simulink model "rx_channelizer_PL"  (R2024a)
settings: Solver=VariableStepAuto  StartTime=0.0  StopTime=num_ch*150/fs  RelTol=1e-3
PreLoadFcn:
  | ch_rate = 41e6; % per channel sample rate
  | num_ch = 32;
  | flip_cnt = num_ch/2 - 1; % flip data count size
  | % 6 coeffs/ch;
  | PLclk=ch_rate*16; % PL clock frequency
  | fs = ch_rate*num_ch;
  | sample_rate = 1/fs;
  | base_freq=1e6; % what base channel frequency to modulate?
  | 
  | generate_prototype_FIR; % create FIR coeffs
undefined symbols (not defined in the file): ch0, ch1, ch10, ch11, ch12, ch13, ch14, ch15, ch16, ch17, ch18, ch19, ch2, ch20, ch21, ch22, ch23, ch24, ch25, ch26, ch27, ch28, ch29, ch3, ch30, ch31, ch4, ch5, ch6, ch7, ch8, ch9, S, vsva2197, xcvc1902
libraries: hdlBasic x69, dspsrcs4 x4, hdlSSR x3, hdlDSPIP x2, dspmlti4 x1, dspxfrm3 x1, vmcUtilities x1
(part 1 of 2)
settings Model: Creator=mmi  LastModifiedBy=robg
settings SolverCC: AlgebraicLoopSolver=TrustRegion
settings DebuggingCC: UnconnectedInputMsg=warning  UnconnectedOutputMsg=warning  UnconnectedLineMsg=warning
settings HardwareCC: ProdBitPerPointer=32  ProdBitPerSizeT=32  ProdBitPerPtrDiffT=32  ProdLargestAtomicFloat=None  ProdIntDivRoundTo=Undefined  ProdEndianess=Unspecified  ProdWordSize=32  ProdHWDeviceType=ASIC/FPGA->ASIC/FPGA  TargetBitPerLong=64  TargetBitPerPointer=64  TargetBitPerSizeT=64  TargetBitPerPtrDiffT=64  TargetLongLongMode=on  TargetIntDivRoundTo=Zero  TargetEndianess=LittleEndian  TargetWordSize=64  TargetHWDeviceType=Custom Processor->MATLAB Host Computer  ProdEqTarget=off
settings ModelReferenceCC: EnableRefExpFcnMdlSchedulingChecks=on
settings RTWCC: GPUComputeCapability=3.5  DLArmComputeVersion=19.05
settings ConfigComp: CovBoundaryAbsTol=1.0e-5

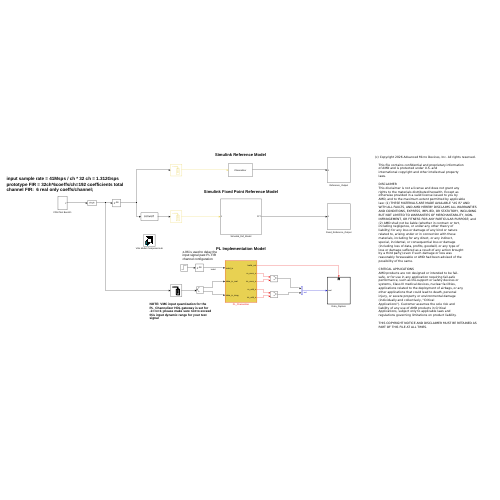
[thumbnail: Simulink's stored preview of the top-level diagram]
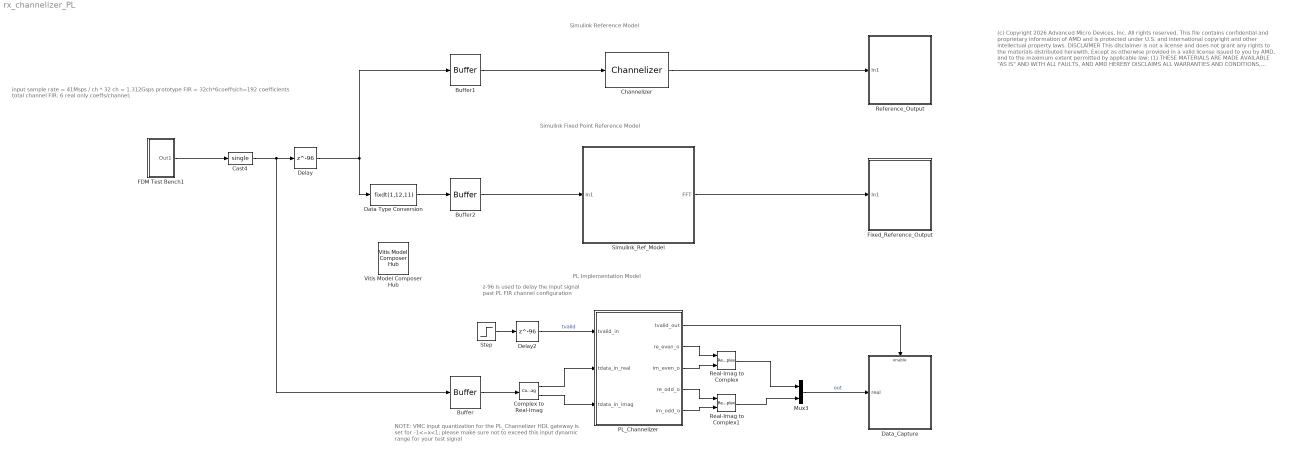
== system rx_channelizer_PL ==
  note: PL Implementation Model
  note: Simulink Fixed Point Reference Model
  note: Simulink Reference Model
  note: z-96 is used to delay the input signal past PL FIR channel configuration
  note: input sample rate = 41Msps / ch * 32 ch = 1.312Gsps
      | prototype FIR = 32ch*6coeffs/ch=192 coefficients total
      | channel FIR: 6 real only coeffs/channel;
  note: NOTE: VMC input quantization for the PL_Channelizer HDL gateway is set for -1<=x<1; please make sure not to exceed this input dynamic range for your test signal
  note: (c) Copyright 2026 Advanced Micro Devices, Inc. All rights reserved.
      |
      | This file contains confidential and proprietary information
      | of AMD and is protected under U.S. and
      | international copyright and other intellectual property
      | laws.
      |
      | DISCLAIMER
      | This disclaimer is not a license and does not grant any
      | rights to the materials distributed herewith. Except as
      | otherwise provided in a valid license issued to you by
      | AMD, and to the maximum extent permitted by applicable
      | law: (1) THESE MATERIALS ARE MADE AVAILABLE "AS IS" AND
      | WITH ALL FAULTS, AND AMD HEREBY DISCLAIMS ALL WARRANTIES
      | AND CONDITIONS, EXPRESS, IMPLIED, OR STATUTORY, INCLUDING
      | BUT NOT LIMITED TO WARRANTIES OF MERCHANTABILITY, NON-
      | INFRINGEMENT, OR FITNESS FOR ANY PARTICULAR PURPOSE; and
      | (2) AMD shall not be liable (whether in contract or tort,
      | including negligence, or under any other theory of
      | liability) for any loss or damage of any kind or nature
      | related to, arising under or in connection with these
      | materials, including for any direct, or any indirect,
      | special, incidental, or consequential loss or damage
      | (including loss of data, profits, goodwill, or any type of
      | loss or damage suffered as a result of any action brought
      | by a third party) even if such damage or loss was
      | reasonably foreseeable or AMD had been advised of the
      | possibility of the same.
      |
      | CRITICAL APPLICATIONS
      | AMD products are not designed or intended to be fail-
      | safe, or for use in any application requiring fail-safe
      | performance, such as life-support or safety devices or
      | systems, Class III medical devices, nuclear facilities,
      | applications related to the deployment of airbags, or any
      | other applications that could lead to death, personal
      | injury, or severe property or environmental damage
      | (individually and collectively, "Critical
      | Applications"). Customer assumes the sole risk and
      | liability of any use of AMD products in Critical
      | Applications, subject only to applicable laws and
      | regulations governing limitations on product liability.
      |
      | THIS COPYRIGHT NOTICE AND DISCLAIMER MUST BE RETAINED AS
      | PART OF THIS FILE AT ALL TIMES.
  Buffer : Buffer  N=2  OutputFrames=off
  Buffer1 : Buffer  N=num_ch*1  OutputFrames=off
  Buffer2 : Buffer  N=num_ch  OutputFrames=off
  Cast4 : DataTypeConversion  OutDataTypeStr=single  SaturateOnIntegerOverflow=off  RndMeth=Floor
  Channelizer : dspmlti4/Channelizer  NumFrequencyBands=32  DecimationFactor=Number of frequency bands  Specification=Coefficients  CoefficientsPort=off  NumTapsPerBand=6  StopbandAttenuation=80  LowpassCoefficients=pf  AllowArbitraryInputLength=off  BandsAsSeparateOutputPorts=off  SimulateUsing=Interpreted execution
  Complex to Real-Imag : ComplexToRealImag
  Data Type Conversion : DataTypeConversion  OutDataTypeStr=fixdt(1,12,11)  SaturateOnIntegerOverflow=off  RndMeth=Floor
  Data_Capture : Subsystem  TreatAsAtomicUnit=on
  Delay : Delay  DelayLength=96
  Delay2 : Delay  DelayLength=96
  FDM Test Bench1 : Subsystem
  Fixed_Reference_Output : Subsystem
  Mux3 : Mux  Inputs=2
  PL_Channelizer : Subsystem
  Real-Imag to Complex : RealImagToComplex
  Real-Imag to Complex1 : RealImagToComplex
  Reference_Output : Subsystem
  Simulink_Ref_Model : Subsystem
  Step : Step  Time=65/(ch_rate*16)  SampleTime=1/(ch_rate*16)
  Vitis Model Composer Hub : vmcUtilities/Vitis Model Composer Hub  Tag=genX  CodeGeneration=off  SubsystemName=PL_Channelizer  BlockHierPath=rx_channelizer_PL/PL_Channelizer  CompilationType=HDLCompilation  SubsystemType=HDLNode  ExportTypeV2=IP Catalog  StartColumn=1  NumberOfColumns=1  TargetDirectory=./netlist_PL  exportDesign=off  analyzeDesign=on  validateDesignOnHw=off  ExportType=AI Engines  IpVendor=xilinx.com  IpLibrary=hls  IpVersion=1.0  IpHWLanguage=Verilog  AieCompilerOptions={}  AieSimulatorOptions={}  CreateTestbench=on  TestbenchStackSize=10  RunRtlSim=off  RunCSim=off  RunAieSim=off  AieSimTimeout=50000  RunAieSimProfiling=off  LaunchVitisAnalyzer=off  PlotOutput=off  RunX86Sim=off  X86SimTimeout=10  GenHwImage=off  GenLibadfXo=on  GenHwValidationCode=off  PlatformType=Not Specified  HwSystemType=Baremetal  HwValidationTarget=hw  ProjDevice=Versal VCK190 Evaluation Platform with New SD Level Shifter (xcvc1902-vsva2197-2MP-e-S)  ProjDevicePart=xcvc1902-vsva2197-2MP-e-S  AIEType=AIE  SamplePeriod=-1  ClockFrequency=200  DataPathParallelism=1  xilinxfamily=versalaicore  part=xcvc1902  speed=-2MP-e-S  package=vsva2197  directory=./netlist_PL/ip/PL_Channelizer/src  testbench=off  incr_netlist=off  synthesis_tool=Vivado  clock_wrapper=Clock Enables  dbl_ovrd=According to Block Masks  dcm_input_clock_period=10  sysclk_period=1e9/PLclk  simulink_period=1/(ch_rate*16)  eval_field=0  IPInfoJsonString="{\"HDLSubsystem\":{\"SubsystemName\":\"PL_Channelizer\",\"IPName\":\"PL_Channelizer\",\"IPLibrary\":\"VMC\",\"IPVendor\":\"User Company\",\"IPVersion\":\"1.0\",\"TargetDirectory\":\"./netlist_PL\",\"SubsystemDir\":\"./netlist_PL/ip/PL_Channelizer\"}}"  LogFileName=/home/mmi/xmc/basics/Channelizer/WTS/netlist_PL/model_composer.log  NThreads=4  IPConfigFile=/tmp/vmctmp-16210593561582334344/rx_channelizer_PL_ipconfig.json
  wires:
  Buffer1/1 -> Channelizer/1
  Delay2/1 -> PL_Channelizer/1(tvalid_in)  "tvalid"
  PL_Channelizer/1(tvalid_out) -> Data_Capture/Enable
  FDM Test Bench1/1(Out1) -> Cast4/1
  Cast4/1 -> Buffer/1, Delay/1
  Delay/1 -> Data Type Conversion/1, Buffer1/1
  Data Type Conversion/1 -> Buffer2/1
  Complex to Real-Imag/1 -> PL_Channelizer/2(tdata_in_real)
  Buffer2/1 -> Simulink_Ref_Model/1(In1)
  Step/1 -> Delay2/1
  Buffer/1 -> Complex to Real-Imag/1
  Complex to Real-Imag/2 -> PL_Channelizer/3(tdata_in_imag)
  Real-Imag to Complex/1 -> Mux3/1
  Mux3/1 -> Data_Capture/1(real)  "out"
  Real-Imag to Complex1/1 -> Mux3/2
  PL_Channelizer/2(re_even_o) -> Real-Imag to Complex/1
  PL_Channelizer/3(im_even_o) -> Real-Imag to Complex/2
  PL_Channelizer/4(re_odd_o) -> Real-Imag to Complex1/1
  PL_Channelizer/5(im_odd_o) -> Real-Imag to Complex1/2
  Simulink_Ref_Model/1(FFT) -> Fixed_Reference_Output/1(In1)
  Channelizer/1 -> Reference_Output/1(In1)

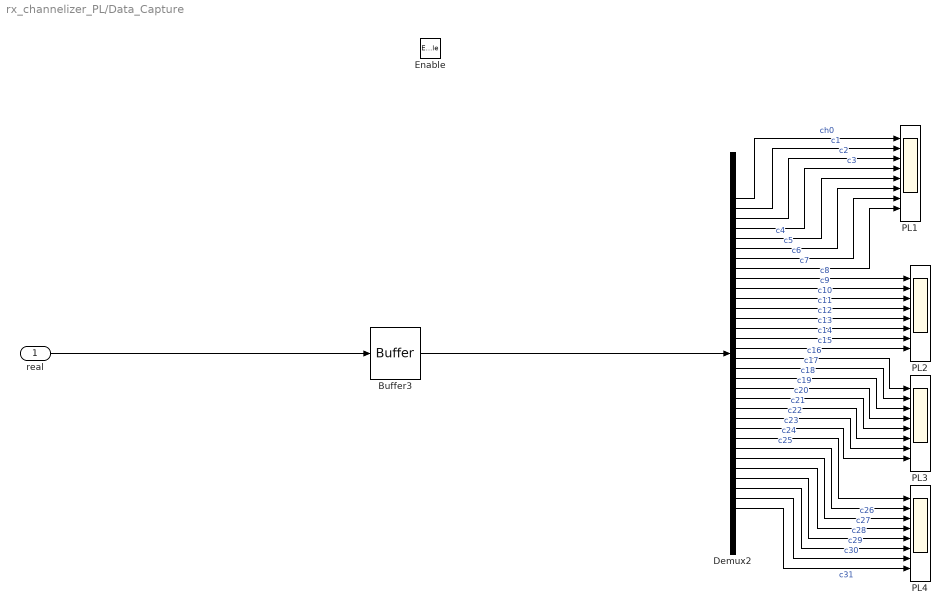
== system rx_channelizer_PL/Data_Capture ==
  real : Inport
  Enable : EnablePort
  Buffer3 : Buffer  N=32  OutputFrames=off
  Demux2 : Demux  Outputs=num_ch
  PL{1..4} (4 alike) : Scope  NumInputPorts=8
  wires:
  Demux2/18 -> PL3/2  "c17"
  Demux2/24 -> PL3/8  "c23"
  Demux2/19 -> PL3/3  "c18"
  Demux2/23 -> PL3/7  "c22"
  Demux2/12 -> PL2/4  "c11"
  Demux2/27 -> PL4/3  "c26"
  Demux2/15 -> PL2/7  "c14"
  Demux2/32 -> PL4/8  "c31"
  Demux2/10 -> PL2/2  "c9"
  Demux2/29 -> PL4/5  "c28"
  Demux2/5 -> PL1/5  "c4"
  Demux2/28 -> PL4/4  "c27"
  Demux2/30 -> PL4/6  "c29"
  Demux2/20 -> PL3/4  "c19"
  Demux2/17 -> PL3/1  "c16"
  Buffer3/1 -> Demux2/1
  Demux2/14 -> PL2/6  "c13"
  Demux2/21 -> PL3/5  "c20"
  Demux2/7 -> PL1/7  "c6"
  Demux2/6 -> PL1/6  "c5"
  Demux2/9 -> PL2/1  "c8"
  Demux2/13 -> PL2/5  "c12"
  Demux2/16 -> PL2/8  "c15"
  Demux2/3 -> PL1/3  "c2"
  Demux2/31 -> PL4/7  "c30"
  Demux2/26 -> PL4/2  "c25"
  Demux2/2 -> PL1/2  "c1"
  Demux2/4 -> PL1/4  "c3"
  Demux2/22 -> PL3/6  "c21"
  Demux2/11 -> PL2/3  "c10"
  Demux2/25 -> PL4/1  "c24"
  Demux2/8 -> PL1/8  "c7"
  Demux2/1 -> PL1/1  "ch0"
  real/1 -> Buffer3/1

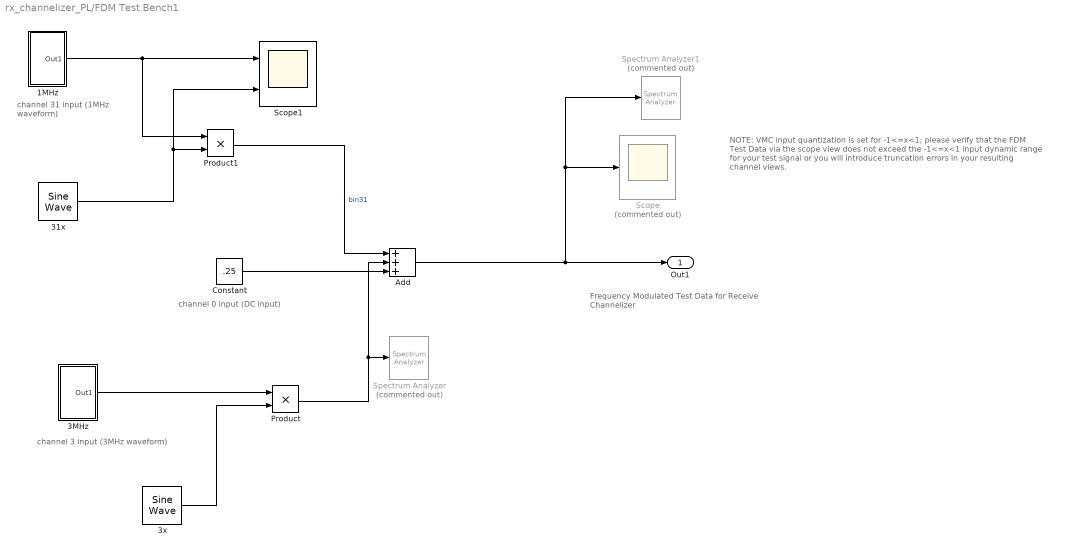
== system rx_channelizer_PL/FDM Test Bench1 ==
  note: Frequency Modulated Test Data for Receive Channelizer
  note: channel 0 input (DC input)
  note: NOTE: VMC input quantization is set for -1<=x<1; please verify that the FDM Test Data via the scope view does not exceed the -1<=x<1 input dynamic range for your test signal or you will introduce truncation errors in your resulting channel views.
  note: channel 31 input (1MHz waveform)
  note: channel 3 input (3MHz waveform)
  1MHz : Subsystem
  31x : dspsrcs4/Sine Wave  Amplitude=0.25  Frequency=31*ch_rate  Phase=0  SampleMode=Discrete  OutComplex=Complex  CompMethod=Trigonometric fcn  TableSize=Speed  SampleTime=sample_rate  SamplesPerFrame=1  ResetState=Restart at time zero  OutputFrames=off  dataType=double  wordLen=16  udDataType=sfix(16)  fracBitsMode=Best precision  numFracBits=15  OutDataTypeStr=double  LastOutDataTypeStr=double
  3MHz : Subsystem
  3x : dspsrcs4/Sine Wave  Amplitude=0.5  Frequency=3*ch_rate  Phase=0  SampleMode=Discrete  OutComplex=Complex  CompMethod=Trigonometric fcn  TableSize=Speed  SampleTime=sample_rate  SamplesPerFrame=1  ResetState=Restart at time zero  OutputFrames=off  dataType=double  wordLen=16  udDataType=sfix(16)  fracBitsMode=Best precision  numFracBits=15  OutDataTypeStr=double  LastOutDataTypeStr=double
  Add : Sum  Inputs=+++
  Constant : Constant  Value=.25
  Product : Product
  Product1 : Product
  Scope : Scope  Commented=on
  Scope1 : Scope  NumInputPorts=2
  Spectrum Analyzer : SpectrumAnalyzer  Commented=on  WindowPosition=[674.000000,677.000000,1237.000000,1149.000000,]  ScopeFrameLocation=window  PlotAsTwoSidedSpectrum=off  Span=656000000  CenterFrequency=328000000  StartFrequency=0  StopFrequency=656000000  YLimits=[-56.29644658,26.27291606]  SelectedToolstripTab=spectrumAnalyzerToolstrip.measurementsTab
  Spectrum Analyzer1 : SpectrumAnalyzer  Commented=on  WindowPosition=[359.000000,185.000000,2081.000000,1202.000000,]  Visible=on  ScopeFrameLocation=window  Span=656000000  CenterFrequency=328000000  StartFrequency=0  StopFrequency=656000000  YLimits=[-50.98624856,25.61945453]  SelectedToolstripTab=spectrumAnalyzerToolstrip.spectrumTab
  Out1 : Outport
  wires:
  3x/1 -> Product/2
  1MHz/1(Out1) -> Product1/1, Scope1/1
  Product1/1 -> Add/1  "bin31"
  Product/1 -> Spectrum Analyzer/1, Add/2
  31x/1 -> Scope1/2, Product1/2
  Constant/1 -> Add/3
  Add/1 -> Spectrum Analyzer1/1, Scope/1, Out1/1
  3MHz/1(Out1) -> Product/1

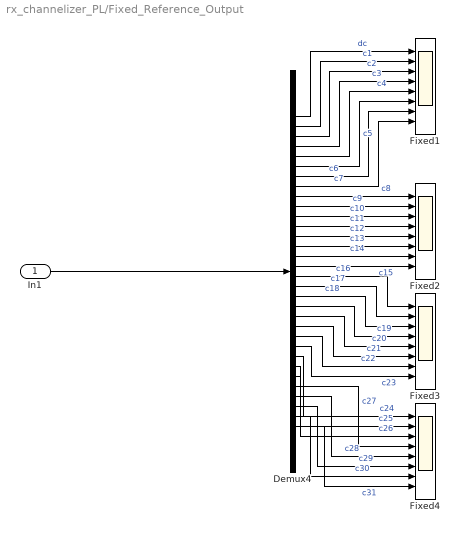
== system rx_channelizer_PL/Fixed_Reference_Output ==
  In1 : Inport
  Demux4 : Demux  Outputs=num_ch
  Fixed{1..4} (4 alike) : Scope  NumInputPorts=8
  wires:
  Demux4/16 -> Fixed2/8  "c15"
  Demux4/29 -> Fixed4/5  "c28"
  Demux4/21 -> Fixed3/5  "c20"
  Demux4/1 -> Fixed1/1  "dc"
  Demux4/17 -> Fixed3/1  "c16"
  Demux4/6 -> Fixed1/6  "c5"
  Demux4/19 -> Fixed3/3  "c18"
  Demux4/30 -> Fixed4/6  "c29"
  Demux4/2 -> Fixed1/2  "c1"
  Demux4/10 -> Fixed2/2  "c9"
  Demux4/32 -> Fixed4/8  "c31"
  Demux4/27 -> Fixed4/3  "c26"
  Demux4/3 -> Fixed1/3  "c2"
  Demux4/22 -> Fixed3/6  "c21"
  Demux4/8 -> Fixed1/8  "c7"
  Demux4/13 -> Fixed2/5  "c12"
  Demux4/5 -> Fixed1/5  "c4"
  In1/1 -> Demux4/1
  Demux4/24 -> Fixed3/8  "c23"
  Demux4/25 -> Fixed4/1  "c24"
  Demux4/12 -> Fixed2/4  "c11"
  Demux4/28 -> Fixed4/4  "c27"
  Demux4/26 -> Fixed4/2  "c25"
  Demux4/31 -> Fixed4/7  "c30"
  Demux4/18 -> Fixed3/2  "c17"
  Demux4/20 -> Fixed3/4  "c19"
  Demux4/9 -> Fixed2/1  "c8"
  Demux4/15 -> Fixed2/7  "c14"
  Demux4/7 -> Fixed1/7  "c6"
  Demux4/14 -> Fixed2/6  "c13"
  Demux4/11 -> Fixed2/3  "c10"
  Demux4/4 -> Fixed1/4  "c3"
  Demux4/23 -> Fixed3/7  "c22"

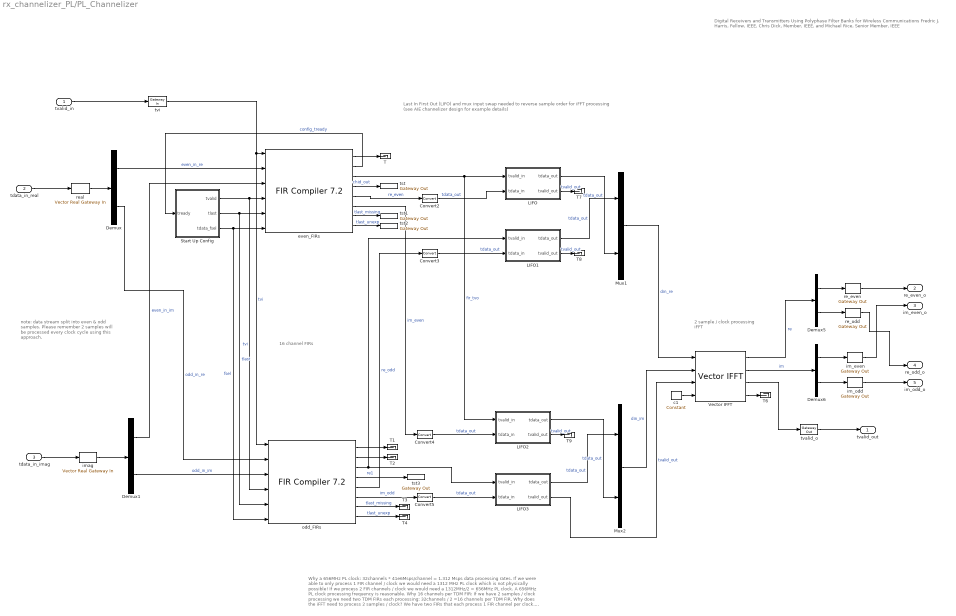
== system rx_channelizer_PL/PL_Channelizer ==
  note: Last In First Out (LIFO) and mux input swap needed to reverse sample order for iFFT processing (see AIE channelizer design for example details)
  note: Why a 656MHz PL clock: 32channels * 41e6Msps/channel = 1.312 Msps data processing rates.
      |
      | If we were able to only process 1 FIR channel / clock we would need a 1312 MHz PL clock which is not physically possible! If we process 2 FIR channels / clock we would need a 1312MHz/2 = 656MHz PL clock. A 656MHz PL clock processing frequency is reasonable.
      |
      | Why 16 channels per TDM FIR:
      | If we have 2 samples / clock processing we need two TDM FIRs each processing: 32channels / 2 =16 channels per TDM FIR.
      |
      | Why does the iFFT need to process 2 samples / clock? We have two FIRs that each process 1 FIR channel per clock. Therefore the FFT also needs to process 2 samples / clock.
  note: 2 sample / clock processing iFFT
  note: 16 channel FIRs
  note: note: data stream split into even & odd samples. Please remember 2 samples will be processed every clock cycle using this approach.
  note: Digital Receivers and Transmitters Using Polyphase
      | Filter Banks for Wireless Communications
      | Fredric J. Harris, Fellow, IEEE, Chris Dick, Member, IEEE, and Michael Rice, Senior Member, IEEE
  tvalid_in : Inport
  tdata_in_real : Inport  Port=2
  tdata_in_imag : Inport  Port=3
  Convert{2..5} (4 alike) : hdlBasic/Convert  gui_display_data_type=Fixed-point  arith_type=Signed (2's comp)  n_bits=23  bin_pt=22  float_type=Single  exp_bits=8  fraction_bits=24  quantization=Truncate  overflow=Wrap  en=off  latency=0  pipeline=off  XmcBlockStatus=1  maskContainerNames=group2  block_type=convert  block_config=sysgen:Convert_config  block_width=595  block_height=885
  Demux{,1,5..6} (4 alike) : Demux  Outputs=2
  LIFO : Subsystem
  LIFO1 : Subsystem
  LIFO2 : Subsystem
  LIFO3 : Subsystem
  Mux1 : Mux  Inputs=2
  Mux2 : Mux  Inputs=2
  Start Up Config : Subsystem
  T{,1..4,6..9} (9 alike) : Terminator
  Vector IFFT : hdlSSR/Vector IFFT  N=num_ch  n_bits=27  bin_pt=22  rounding=on  bypass_input_swap=off  bypass_ouput_dsn=off  bram_threshold=258  use_cm4=3  use_cb=off  sg_ssr=2  block_type=ifft_ssr  W_high=1  W_low=-17  XmcBlockStatus=1  sg_ssr_prev=2  maskContainerNames=group3
  c1 : hdlBasic/Constant  const=0  gui_display_data_type=Fixed-point  arith_type=Unsigned  n_bits=log2(num_ch)  bin_pt=0  preci_type=Single  exp_width=8  frac_width=24  explicit_period=on  period=1/(ch_rate*16)  XmcBlockStatus=1  maskContainerNames=tabcontainer1  block_type=constant  block_config=sysgen:Constant_config
  even_FIRs : hdlDSPIP/FIR Compiler 7.2   coefficientvector=[ ch31 ch29 ch27 ch25 ch23 ch21 ch19 ch17 ch15 ch13 ch11 ch9 ch7 ch5 ch3 ch1 ]  coefficient_sets=16  coefficient_reload=off  filter_type=Single_Rate  rate_change_type=Integer  interpolation_rate=1  decimation_rate=1  zero_pack_factor=1  channel_sequence=Basic  number_channels=16  pattern_list='P4-0,P4-1,P4-2,P4-3,P4-4'  number_paths=2  ratespecification=Input_Sample_Period  sampleperiod=1  hardwareoversamplingrate=1  coefficient_sign=Unsigned  quantization=Quantize_Only  coefficient_width=18  bestprecision=on  coefficient_fractional_bits=22  coefficient_structure=Inferred  output_rounding_mode=Truncate_LSBs  output_width=24  filter_architecture=Systolic_Multiply_Accumulate  optimization_goal=Area  optimization_list='None'  data_buffer_type=Automatic  coefficient_buffer_type=Automatic  input_buffer_type=Automatic  output_buffer_type=Automatic  preference_for_other_storage=Automatic  multi_column_support=Automatic  columnconfig='6'  inter_column_pipe_length=4  data_has_tlast=Not_Required  m_data_has_tready=off  s_data_has_fifo=off  s_data_has_tuser=Not_Required  m_data_has_tuser=Chan_ID_Field  s_config_sync_mode=On_Vector  s_config_method=By_Channel  num_reload_slots=1  has_aclken=off  has_aresetn=off  reset_data_vector=on  trim_axipin_name=on  simulation_type=xsim  simulation_model=sysgen:xfirv7_2_cmodel  data_path_portlist={ 's_axis_data_tdata', 'm_axis_data_tdata' }  passband_min=0.0  passband_max=0.5  stopband_min=0.5  stopband_max=1.0  filter_selection=1  gui_behaviour='Sysgen_GUI'  data_sign=Signed  data_width=16  data_fractional_bits=0  data_tuser_width=1  wrapper_available=true  ip_wrap_arbitrary_binary_point=true  ip_name=FIR Compiler  ip_version=7.2  dsptool_ready=true  ipcore_usecache=true  ipcore_useipmodelcache=true  port_translation_map={ 'aclken' => 'en', 'aresetn' => 'rst' }  run_core_at_system_period=true  ipcore_xco_need_fpga_part=true  ipcore_fpga_part=[]  XmcBlockStatus=1  maskContainerNames=tabcontainer1  block_type=fir_compiler_v7_2  block_config=sysgen:rodinimport_config  block_width=820  block_height=600
  im_even : hdlBasic/Gateway Out  inherit_from_input=off  bool_to_boolean=off  hdl_port=on  rows=1  columns=1  UseAsDAC=off  DACChannel='1'  interface=None  automatic_assignment=on  address_offset=hex2dec('00')  intf_name=''  intf_description=''  timing_constraint=None  locs_specified=off  LOCs={}  io_standard={}  XmcBlockStatus=1  maskContainerNames=group4  block_type=gatewayout  block_config=sysgen:gateway_out_config  block_width_w=590  block_height_w=620  block_width=620  block_height=750
  im_odd : hdlBasic/Gateway Out  inherit_from_input=off  bool_to_boolean=off  hdl_port=on  rows=1  columns=1  UseAsDAC=off  DACChannel='1'  interface=None  automatic_assignment=on  address_offset=hex2dec('00')  intf_name=''  intf_description=''  timing_constraint=None  locs_specified=off  LOCs={}  io_standard={}  XmcBlockStatus=1  maskContainerNames=group4  block_type=gatewayout  block_config=sysgen:gateway_out_config  block_width_w=590  block_height_w=620  block_width=620  block_height=750
  imag : hdlSSR/Vector Real Gateway In  gui_display_data_type=Fixed-point  arith_type=Signed (2's comp)  n_bits=12  bin_pt=11  preci_type=Single  exp_width=8  frac_width=24  quantization=Truncate  overflow=Wrap  period=1/(ch_rate*16)  sg_ssr=2  UseAsADC=off  ADCChannel='1'  interface=None  automatic_assignment=on  address_offset=hex2dec('00')  intf_name=''  intf_description=''  default_value=0  timing_constraint=None  locs_specified=off  LOCs={}  io_standard={}  inherit_from_input=off  hdl_port=on  interface_prev=1  block_type=realgatewayin_ssr  XmcBlockStatus=1  sg_ssr_prev=2  maskContainerNames=group4  block_width_w=590  block_height_w=670  block_width=640  block_height=850
  odd_FIRs : hdlDSPIP/FIR Compiler 7.2   coefficientvector="[ ch30 ch28 ch26 ch24 ch22 ch20 ch18 ch16 ch14 ch12 ch10 ch8 ch6 ch4 ch2 ch0  ]"  coefficient_sets=16  coefficient_reload=off  filter_type=Single_Rate  rate_change_type=Integer  interpolation_rate=1  decimation_rate=1  zero_pack_factor=1  channel_sequence=Basic  number_channels=16  pattern_list='P4-0,P4-1,P4-2,P4-3,P4-4'  number_paths=2  ratespecification=Input_Sample_Period  sampleperiod=1  hardwareoversamplingrate=1  coefficient_sign=Unsigned  quantization=Quantize_Only  coefficient_width=18  bestprecision=on  coefficient_fractional_bits=22  coefficient_structure=Inferred  output_rounding_mode=Truncate_LSBs  output_width=24  filter_architecture=Systolic_Multiply_Accumulate  optimization_goal=Area  optimization_list='None'  data_buffer_type=Automatic  coefficient_buffer_type=Automatic  input_buffer_type=Automatic  output_buffer_type=Automatic  preference_for_other_storage=Automatic  multi_column_support=Automatic  columnconfig='6'  inter_column_pipe_length=4  data_has_tlast=Not_Required  m_data_has_tready=off  s_data_has_fifo=off  s_data_has_tuser=Not_Required  m_data_has_tuser=Chan_ID_Field  s_config_sync_mode=On_Vector  s_config_method=By_Channel  num_reload_slots=1  has_aclken=off  has_aresetn=off  reset_data_vector=on  trim_axipin_name=on  simulation_type=xsim  simulation_model=sysgen:xfirv7_2_cmodel  data_path_portlist={ 's_axis_data_tdata', 'm_axis_data_tdata' }  passband_min=0.0  passband_max=0.5  stopband_min=0.5  stopband_max=1.0  filter_selection=1  gui_behaviour='Sysgen_GUI'  data_sign=Signed  data_width=16  data_fractional_bits=0  data_tuser_width=1  wrapper_available=true  ip_wrap_arbitrary_binary_point=true  ip_name=FIR Compiler  ip_version=7.2  dsptool_ready=true  ipcore_usecache=true  ipcore_useipmodelcache=true  port_translation_map={ 'aclken' => 'en', 'aresetn' => 'rst' }  run_core_at_system_period=true  ipcore_xco_need_fpga_part=true  ipcore_fpga_part=[]  XmcBlockStatus=1  maskContainerNames=tabcontainer1  block_type=fir_compiler_v7_2  block_config=sysgen:rodinimport_config  block_width=820  block_height=600
  re_even : hdlBasic/Gateway Out  inherit_from_input=off  bool_to_boolean=off  hdl_port=on  rows=1  columns=1  UseAsDAC=off  DACChannel='1'  interface=None  automatic_assignment=on  address_offset=hex2dec('00')  intf_name=''  intf_description=''  timing_constraint=None  locs_specified=off  LOCs={}  io_standard={}  XmcBlockStatus=1  maskContainerNames=group4  block_type=gatewayout  block_config=sysgen:gateway_out_config  block_width_w=590  block_height_w=620  block_width=620  block_height=750
  re_odd : hdlBasic/Gateway Out  inherit_from_input=off  bool_to_boolean=off  hdl_port=on  rows=1  columns=1  UseAsDAC=off  DACChannel='1'  interface=None  automatic_assignment=on  address_offset=hex2dec('00')  intf_name=''  intf_description=''  timing_constraint=None  locs_specified=off  LOCs={}  io_standard={}  XmcBlockStatus=1  maskContainerNames=group4  block_type=gatewayout  block_config=sysgen:gateway_out_config  block_width_w=590  block_height_w=620  block_width=620  block_height=750
  real : hdlSSR/Vector Real Gateway In  gui_display_data_type=Fixed-point  arith_type=Signed (2's comp)  n_bits=12  bin_pt=11  preci_type=Single  exp_width=8  frac_width=24  quantization=Truncate  overflow=Wrap  period=1/(ch_rate*16)  sg_ssr=2  UseAsADC=off  ADCChannel='1'  interface=None  automatic_assignment=on  address_offset=hex2dec('00')  intf_name=''  intf_description=''  default_value=0  timing_constraint=None  locs_specified=off  LOCs={}  io_standard={}  inherit_from_input=off  hdl_port=on  interface_prev=1  block_type=realgatewayin_ssr  XmcBlockStatus=1  sg_ssr_prev=2  maskContainerNames=group4  block_width_w=590  block_height_w=670  block_width=640  block_height=850
  tst{,1..3} (4 alike) : hdlBasic/Gateway Out  inherit_from_input=off  bool_to_boolean=off  hdl_port=off  rows=1  columns=1  UseAsDAC=off  DACChannel='1'  interface=None  automatic_assignment=on  address_offset=hex2dec('00')  intf_name=''  intf_description=''  timing_constraint=None  locs_specified=off  LOCs={}  io_standard={}  XmcBlockStatus=1  maskContainerNames=group4  block_type=gatewayout  block_config=sysgen:gateway_out_config  block_width_w=590  block_height_w=620  block_width=620  block_height=750
  tvalid_o : hdlBasic/Gateway Out  inherit_from_input=off  bool_to_boolean=off  hdl_port=on  rows=1  columns=1  UseAsDAC=off  DACChannel='1'  interface=None  automatic_assignment=on  address_offset=hex2dec('00')  intf_name=''  intf_description=''  timing_constraint=None  locs_specified=off  LOCs={}  io_standard={}  XmcBlockStatus=1  maskContainerNames=group4  block_type=gatewayout  block_config=sysgen:gateway_out_config  block_width_w=590  block_height_w=620  block_width=620  block_height=750
  tvi : hdlBasic/Gateway In  gui_display_data_type=Boolean  arith_type=Boolean  n_bits=12  bin_pt=0  preci_type=Single  exp_width=8  frac_width=24  rows=1  columns=1  quantization=Truncate  overflow=Wrap  period=1/(ch_rate*16)  UseAsADC=off  ADCChannel='1'  interface=None  automatic_assignment=on  address_offset=hex2dec('00')  intf_name=''  intf_description=''  default_value=0  timing_constraint=None  locs_specified=off  LOCs={}  io_standard={}  inherit_from_input=off  hdl_port=on  XmcBlockStatus=1  maskContainerNames=group4  block_type=gatewayin  block_config=sysgen:gateway_in_config  block_width_w=590  block_height_w=620  block_width=640  block_height=850
  tvalid_out : Outport
  re_even_o : Outport  Port=2
  im_even_o : Outport  Port=3
  re_odd_o : Outport  Port=4
  im_odd_o : Outport  Port=5
  wires:
  odd_FIRs/1 -> T1/1
  odd_FIRs/4 -> tst3/1  "re1"
  tvi/1 -> odd_FIRs/1, even_FIRs/1  "tvi"
  Demux1/2 -> odd_FIRs/3  "odd_in_im"
  even_FIRs/3 -> LIFO2/1(tvalid_in), LIFO/1(tvalid_in)  "fir_tvo"
  odd_FIRs/6 -> Convert5/1  "im_odd"
  Start Up Config/3(tdata_fsel) -> odd_FIRs/6, even_FIRs/6  "fsel"
  tvalid_in/1 -> tvi/1
  even_FIRs/2 -> Start Up Config/1(tready)  "config_tready"
  even_FIRs/6 -> Convert4/1  "im_even"
  odd_FIRs/7 -> T3/1  "tlast_missing"
  Start Up Config/1(tvalid) -> odd_FIRs/4, even_FIRs/4  "tvi"
  even_FIRs/8 -> tst2/1  "tlast_unexp"
  even_FIRs/5 -> Convert2/1  "re_even"
  Demux/1 -> even_FIRs/2  "even_in_re"
  Demux1/1 -> even_FIRs/3  "even_in_im"
  odd_FIRs/8 -> T4/1  "tlast_unexp"
  Mux1/1 -> Vector IFFT/1  "din_re"
  odd_FIRs/5 -> Convert3/1  "re_odd"
  Start Up Config/2(tlast) -> odd_FIRs/5, even_FIRs/5  "tlast"
  even_FIRs/1 -> T/1
  odd_FIRs/2 -> T2/1
  even_FIRs/4 -> tst/1  "chid_out"
  even_FIRs/7 -> tst1/1  "tlast_missing"
  Demux/2 -> odd_FIRs/2  "odd_in_re"
  Vector IFFT/1 -> Demux5/1  "re"
  Vector IFFT/2 -> Demux6/1  "im"
  re_odd/1 -> re_odd_o/1
  re_even/1 -> re_even_o/1
  im_odd/1 -> im_odd_o/1
  im_even/1 -> im_even_o/1
  Vector IFFT/3 -> tvalid_o/1
  Convert2/1 -> LIFO/2(tdata_in)  "tdata_out"
  Convert3/1 -> LIFO1/2(tdata_in)  "tdata_out"
  Convert4/1 -> LIFO2/2(tdata_in)  "tdata_out"
  odd_FIRs/3 -> LIFO1/1(tvalid_in), LIFO3/1(tvalid_in)
  Demux5/1 -> re_even/1
  Demux5/2 -> re_odd/1
  Demux6/1 -> im_even/1
  Demux6/2 -> im_odd/1
  tdata_in_real/1 -> real/1
  c1/1 -> Vector IFFT/4
  Vector IFFT/4 -> T6/1
  LIFO/2(tvalid_out) -> T7/1  "tvalid_out"
  Mux2/1 -> Vector IFFT/2  "din_im"
  LIFO/1(tdata_out) -> Mux1/2  "tdata_out"
  LIFO1/1(tdata_out) -> Mux1/1  "tdata_out"
  LIFO2/1(tdata_out) -> Mux2/2  "tdata_out"
  Convert5/1 -> LIFO3/2(tdata_in)  "tdata_out"
  LIFO3/1(tdata_out) -> Mux2/1  "tdata_out"
  LIFO3/2(tvalid_out) -> Vector IFFT/3  "tvalid_out"
  LIFO1/2(tvalid_out) -> T8/1  "tvalid_out"
  LIFO2/2(tvalid_out) -> T9/1  "tvalid_out"
  tdata_in_imag/1 -> imag/1
  imag/1 -> Demux1/1
  real/1 -> Demux/1
  tvalid_o/1 -> tvalid_out/1

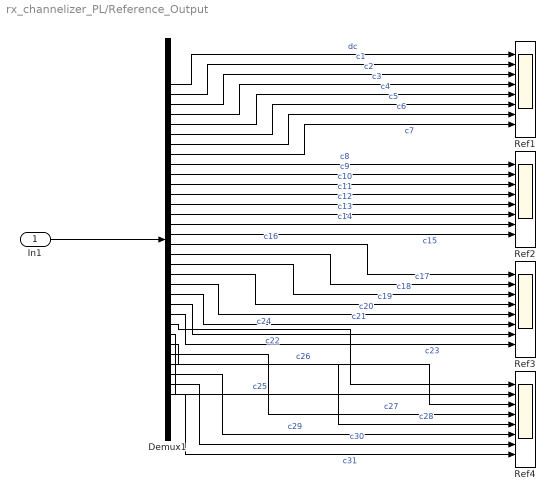
== system rx_channelizer_PL/Reference_Output ==
  In1 : Inport
  Demux1 : Demux  Outputs=num_ch
  Ref{1..4} (4 alike) : Scope  NumInputPorts=8
  wires:
  Demux1/21 -> Ref3/5  "c20"
  Demux1/19 -> Ref3/3  "c18"
  Demux1/32 -> Ref4/8  "c31"
  Demux1/20 -> Ref3/4  "c19"
  Demux1/18 -> Ref3/2  "c17"
  Demux1/11 -> Ref2/3  "c10"
  Demux1/10 -> Ref2/2  "c9"
  Demux1/12 -> Ref2/4  "c11"
  Demux1/13 -> Ref2/5  "c12"
  Demux1/28 -> Ref4/4  "c27"
  Demux1/7 -> Ref1/7  "c6"
  Demux1/14 -> Ref2/6  "c13"
  Demux1/27 -> Ref4/3  "c26"
  Demux1/9 -> Ref2/1  "c8"
  Demux1/16 -> Ref2/8  "c15"
  Demux1/29 -> Ref4/5  "c28"
  Demux1/6 -> Ref1/6  "c5"
  Demux1/26 -> Ref4/2  "c25"
  Demux1/1 -> Ref1/1  "dc"
  Demux1/5 -> Ref1/5  "c4"
  In1/1 -> Demux1/1
  Demux1/3 -> Ref1/3  "c2"
  Demux1/4 -> Ref1/4  "c3"
  Demux1/25 -> Ref4/1  "c24"
  Demux1/31 -> Ref4/7  "c30"
  Demux1/17 -> Ref3/1  "c16"
  Demux1/30 -> Ref4/6  "c29"
  Demux1/8 -> Ref1/8  "c7"
  Demux1/15 -> Ref2/7  "c14"
  Demux1/22 -> Ref3/6  "c21"
  Demux1/2 -> Ref1/2  "c1"
  Demux1/24 -> Ref3/8  "c23"
  Demux1/23 -> Ref3/7  "c22"

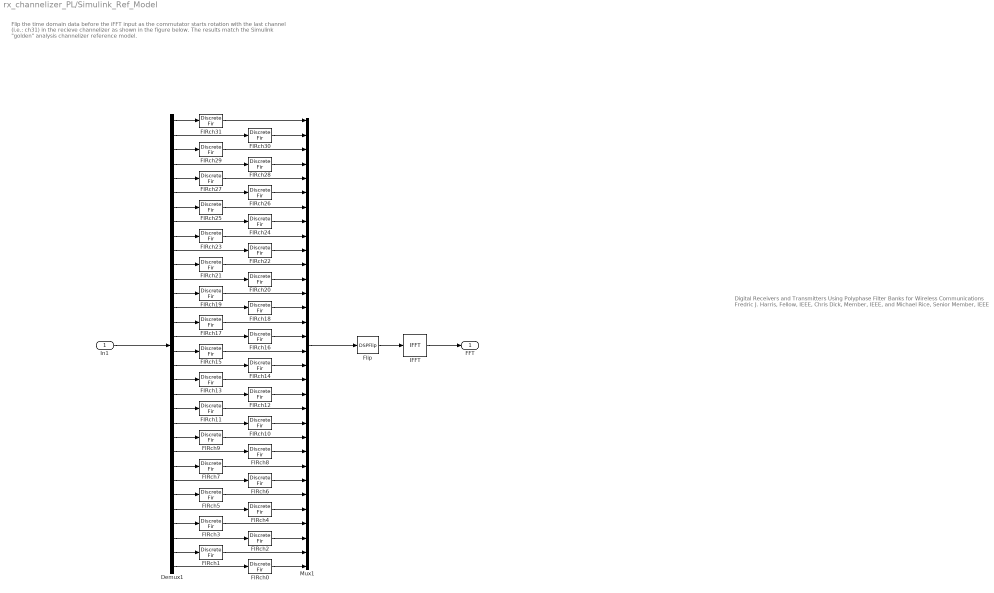
== system rx_channelizer_PL/Simulink_Ref_Model ==
  note: Digital Receivers and Transmitters Using Polyphase
      | Filter Banks for Wireless Communications
      | Fredric J. Harris, Fellow, IEEE, Chris Dick, Member, IEEE, and Michael Rice, Senior Member, IEEE
  note: Flip the time domain data before the iFFT input as the commutator starts rotation with the last channel (i.e.: ch31) in the recieve channelizer as shown in the figure below.
      |
      | The results match the Simulink "golden" analysis channelizer reference model.
  In1 : Inport
  Demux1 : Demux  Outputs=num_ch
  FIRch0 : DiscreteFir  Coefficients=[ch0]  InputProcessing=Columns as channels (frame based)  CoefDataTypeStr=fixdt(1,18,18)  OutDataTypeStr=fixdt(1,23,22)  RndMeth=Convergent
  FIRch1 : DiscreteFir  Coefficients=[ch1]  InputProcessing=Columns as channels (frame based)  CoefDataTypeStr=fixdt(1,18,18)  OutDataTypeStr=fixdt(1,23,22)  RndMeth=Convergent
  FIRch10 : DiscreteFir  Coefficients=[ch10]  InputProcessing=Columns as channels (frame based)  CoefDataTypeStr=fixdt(1,18,18)  OutDataTypeStr=fixdt(1,23,22)  RndMeth=Convergent
  FIRch11 : DiscreteFir  Coefficients=[ch11]  InputProcessing=Columns as channels (frame based)  CoefDataTypeStr=fixdt(1,18,18)  OutDataTypeStr=fixdt(1,23,22)  RndMeth=Convergent
  FIRch12 : DiscreteFir  Coefficients=[ch12]  InputProcessing=Columns as channels (frame based)  CoefDataTypeStr=fixdt(1,18,18)  OutDataTypeStr=fixdt(1,23,22)  RndMeth=Convergent
  FIRch13 : DiscreteFir  Coefficients=[ch13]  InputProcessing=Columns as channels (frame based)  CoefDataTypeStr=fixdt(1,18,18)  OutDataTypeStr=fixdt(1,23,22)  RndMeth=Convergent
  FIRch14 : DiscreteFir  Coefficients=[ch14]  InputProcessing=Columns as channels (frame based)  CoefDataTypeStr=fixdt(1,18,18)  OutDataTypeStr=fixdt(1,23,22)  RndMeth=Convergent
  FIRch15 : DiscreteFir  Coefficients=[ch15]  InputProcessing=Columns as channels (frame based)  CoefDataTypeStr=fixdt(1,18,18)  OutDataTypeStr=fixdt(1,23,22)  RndMeth=Convergent
  FIRch16 : DiscreteFir  Coefficients=[ch16]  InputProcessing=Columns as channels (frame based)  CoefDataTypeStr=fixdt(1,18,18)  OutDataTypeStr=fixdt(1,23,22)  RndMeth=Convergent
  FIRch17 : DiscreteFir  Coefficients=[ch17]  InputProcessing=Columns as channels (frame based)  CoefDataTypeStr=fixdt(1,18,18)  OutDataTypeStr=fixdt(1,23,22)  RndMeth=Convergent
  FIRch18 : DiscreteFir  Coefficients=[ch18]  InputProcessing=Columns as channels (frame based)  CoefDataTypeStr=fixdt(1,18,18)  OutDataTypeStr=fixdt(1,23,22)  RndMeth=Convergent
  FIRch19 : DiscreteFir  Coefficients=[ch19]  InputProcessing=Columns as channels (frame based)  CoefDataTypeStr=fixdt(1,18,18)  OutDataTypeStr=fixdt(1,23,22)  RndMeth=Convergent
  FIRch2 : DiscreteFir  Coefficients=[ch2]  InputProcessing=Columns as channels (frame based)  CoefDataTypeStr=fixdt(1,18,18)  OutDataTypeStr=fixdt(1,23,22)  RndMeth=Convergent
  FIRch20 : DiscreteFir  Coefficients=[ch20]  InputProcessing=Columns as channels (frame based)  CoefDataTypeStr=fixdt(1,18,18)  OutDataTypeStr=fixdt(1,23,22)  RndMeth=Convergent
  FIRch21 : DiscreteFir  Coefficients=[ch21]  InputProcessing=Columns as channels (frame based)  CoefDataTypeStr=fixdt(1,18,18)  OutDataTypeStr=fixdt(1,23,22)  RndMeth=Convergent
  FIRch22 : DiscreteFir  Coefficients=[ch22]  InputProcessing=Columns as channels (frame based)  CoefDataTypeStr=fixdt(1,18,18)  OutDataTypeStr=fixdt(1,23,22)  RndMeth=Convergent
  FIRch23 : DiscreteFir  Coefficients=[ch23]  InputProcessing=Columns as channels (frame based)  CoefDataTypeStr=fixdt(1,18,18)  OutDataTypeStr=fixdt(1,23,22)  RndMeth=Convergent
  FIRch24 : DiscreteFir  Coefficients=[ch24]  InputProcessing=Columns as channels (frame based)  CoefDataTypeStr=fixdt(1,18,18)  OutDataTypeStr=fixdt(1,23,22)  RndMeth=Convergent
  FIRch25 : DiscreteFir  Coefficients=[ch25]  InputProcessing=Columns as channels (frame based)  CoefDataTypeStr=fixdt(1,18,18)  OutDataTypeStr=fixdt(1,23,22)  RndMeth=Convergent
  FIRch26 : DiscreteFir  Coefficients=[ch26]  InputProcessing=Columns as channels (frame based)  CoefDataTypeStr=fixdt(1,18,18)  OutDataTypeStr=fixdt(1,23,22)  RndMeth=Convergent
  FIRch27 : DiscreteFir  Coefficients=[ch27]  InputProcessing=Columns as channels (frame based)  CoefDataTypeStr=fixdt(1,18,18)  OutDataTypeStr=fixdt(1,23,22)  RndMeth=Convergent
  FIRch28 : DiscreteFir  Coefficients=[ch28]  InputProcessing=Columns as channels (frame based)  CoefDataTypeStr=fixdt(1,18,18)  OutDataTypeStr=fixdt(1,23,22)  RndMeth=Convergent
  FIRch29 : DiscreteFir  Coefficients=[ch29]  InputProcessing=Columns as channels (frame based)  CoefDataTypeStr=fixdt(1,18,18)  OutDataTypeStr=fixdt(1,23,22)  RndMeth=Convergent
  FIRch3 : DiscreteFir  Coefficients=[ch3]  InputProcessing=Columns as channels (frame based)  CoefDataTypeStr=fixdt(1,18,18)  OutDataTypeStr=fixdt(1,23,22)  RndMeth=Convergent
  FIRch30 : DiscreteFir  Coefficients=[ch30]  InputProcessing=Columns as channels (frame based)  CoefDataTypeStr=fixdt(1,18,18)  OutDataTypeStr=fixdt(1,23,22)  RndMeth=Convergent
  FIRch31 : DiscreteFir  Coefficients=[ch31]  InputProcessing=Columns as channels (frame based)  CoefDataTypeStr=fixdt(1,18,18)  OutDataTypeStr=fixdt(1,23,22)  RndMeth=Convergent
  FIRch4 : DiscreteFir  Coefficients=[ch4]  InputProcessing=Columns as channels (frame based)  CoefDataTypeStr=fixdt(1,18,18)  OutDataTypeStr=fixdt(1,23,22)  RndMeth=Convergent
  FIRch5 : DiscreteFir  Coefficients=[ch5]  InputProcessing=Columns as channels (frame based)  CoefDataTypeStr=fixdt(1,18,18)  OutDataTypeStr=fixdt(1,23,22)  RndMeth=Convergent
  FIRch6 : DiscreteFir  Coefficients=[ch6]  InputProcessing=Columns as channels (frame based)  CoefDataTypeStr=fixdt(1,18,18)  OutDataTypeStr=fixdt(1,23,22)  RndMeth=Convergent
  FIRch7 : DiscreteFir  Coefficients=[ch7]  InputProcessing=Columns as channels (frame based)  CoefDataTypeStr=fixdt(1,18,18)  OutDataTypeStr=fixdt(1,23,22)  RndMeth=Convergent
  FIRch8 : DiscreteFir  Coefficients=[ch8]  InputProcessing=Columns as channels (frame based)  CoefDataTypeStr=fixdt(1,18,18)  OutDataTypeStr=fixdt(1,23,22)  RndMeth=Convergent
  FIRch9 : DiscreteFir  Coefficients=[ch9]  InputProcessing=Columns as channels (frame based)  CoefDataTypeStr=fixdt(1,18,18)  OutDataTypeStr=fixdt(1,23,22)  RndMeth=Convergent
  Flip : DSPFlip
  IFFT : dspxfrm3/IFFT  FFTImplementation=Auto  CompMethod=Table lookup  TableOpt=NEW  TableOptActive=Speed  BitRevOrder=off  cs_in=off  Normalize=off  InheritFFTLength=on  FFTLength=64  WrapInput=on  mode=Real  outSamplingMode=Sample based  roundingMode=Ceiling  overflowMode=off  firstCoeffDataTypeStr=Inherit: Same word length as input  firstCoeffLastDataTypeStr=Inherit: Same word length as input  outputMin=[]  outputMax=[]
  Mux1 : Mux  Inputs=num_ch
  FFT : Outport
  wires:
  In1/1 -> Demux1/1
  Demux1/1 -> FIRch31/1
  FIRch31/1 -> Mux1/1
  Demux1/2 -> FIRch30/1
  FIRch30/1 -> Mux1/2
  Demux1/3 -> FIRch29/1
  FIRch29/1 -> Mux1/3
  Demux1/4 -> FIRch28/1
  FIRch28/1 -> Mux1/4
  Demux1/5 -> FIRch27/1
  FIRch27/1 -> Mux1/5
  FIRch26/1 -> Mux1/6
  Demux1/6 -> FIRch26/1
  Demux1/7 -> FIRch25/1
  FIRch25/1 -> Mux1/7
  FIRch24/1 -> Mux1/8
  Demux1/8 -> FIRch24/1
  Demux1/9 -> FIRch23/1
  FIRch23/1 -> Mux1/9
  FIRch22/1 -> Mux1/10
  Demux1/10 -> FIRch22/1
  Demux1/11 -> FIRch21/1
  FIRch21/1 -> Mux1/11
  FIRch20/1 -> Mux1/12
  Demux1/12 -> FIRch20/1
  FIRch19/1 -> Mux1/13
  Demux1/13 -> FIRch19/1
  FIRch18/1 -> Mux1/14
  Demux1/14 -> FIRch18/1
  Demux1/15 -> FIRch17/1
  FIRch17/1 -> Mux1/15
  Demux1/16 -> FIRch16/1
  Demux1/17 -> FIRch15/1
  Demux1/18 -> FIRch14/1
  Demux1/19 -> FIRch13/1
  Demux1/20 -> FIRch12/1
  Demux1/21 -> FIRch11/1
  Demux1/22 -> FIRch10/1
  Demux1/23 -> FIRch9/1
  Demux1/24 -> FIRch8/1
  Demux1/25 -> FIRch7/1
  Demux1/26 -> FIRch6/1
  Demux1/27 -> FIRch5/1
  Demux1/28 -> FIRch4/1
  Demux1/29 -> FIRch3/1
  Demux1/30 -> FIRch2/1
  Demux1/31 -> FIRch1/1
  Demux1/32 -> FIRch0/1
  FIRch16/1 -> Mux1/16
  FIRch15/1 -> Mux1/17
  FIRch14/1 -> Mux1/18
  FIRch13/1 -> Mux1/19
  FIRch12/1 -> Mux1/20
  FIRch11/1 -> Mux1/21
  FIRch10/1 -> Mux1/22
  FIRch9/1 -> Mux1/23
  FIRch8/1 -> Mux1/24
  FIRch7/1 -> Mux1/25
  FIRch6/1 -> Mux1/26
  FIRch5/1 -> Mux1/27
  FIRch4/1 -> Mux1/28
  FIRch3/1 -> Mux1/29
  FIRch2/1 -> Mux1/30
  FIRch1/1 -> Mux1/31
  FIRch0/1 -> Mux1/32
  IFFT/1 -> FFT/1
  Mux1/1 -> Flip/1
  Flip/1 -> IFFT/1

== system rx_channelizer_PL/FDM Test Bench1/1MHz ==
  1MHz : dspsrcs4/Sine Wave  Amplitude=0.5  Frequency=base_freq  Phase=0  SampleMode=Discrete  OutComplex=Complex  CompMethod=Trigonometric fcn  TableSize=Speed  SampleTime=sample_rate  SamplesPerFrame=1  ResetState=Restart at time zero  OutputFrames=off  dataType=double  wordLen=16  udDataType=sfix(16)  fracBitsMode=Best precision  numFracBits=15  OutDataTypeStr=double  LastOutDataTypeStr=double
  Out1 : Outport
  wires:
  1MHz/1 -> Out1/1

== system rx_channelizer_PL/FDM Test Bench1/3MHz ==
  3MHz : dspsrcs4/Sine Wave  Amplitude=0.5  Frequency=base_freq*3  Phase=0  SampleMode=Discrete  OutComplex=Complex  CompMethod=Trigonometric fcn  TableSize=Speed  SampleTime=sample_rate  SamplesPerFrame=1  ResetState=Restart at time zero  OutputFrames=off  dataType=double  wordLen=16  udDataType=sfix(16)  fracBitsMode=Best precision  numFracBits=15  OutDataTypeStr=double  LastOutDataTypeStr=double
  Out1 : Outport
  wires:
  3MHz/1 -> Out1/1

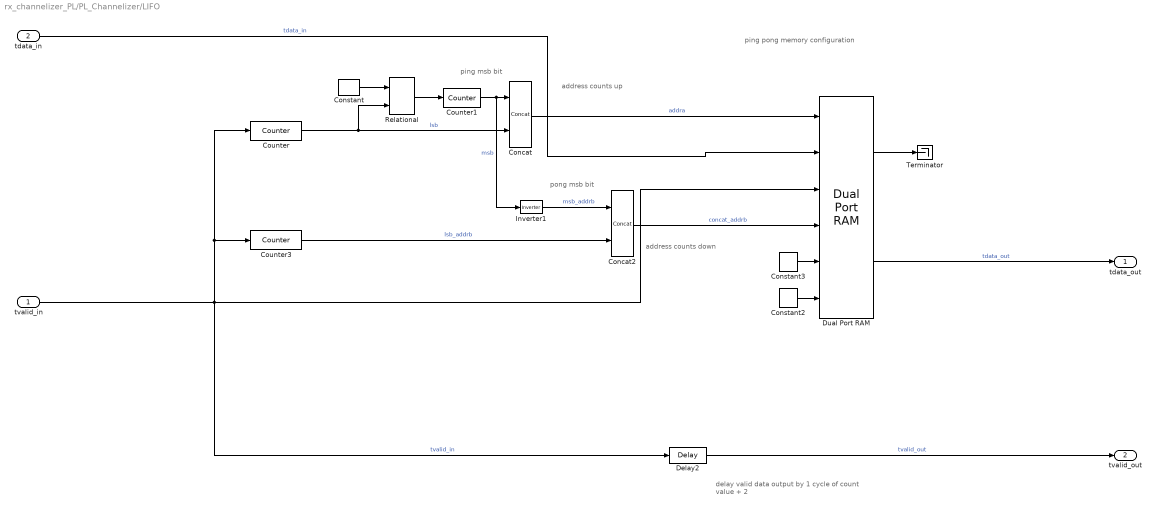
== system rx_channelizer_PL/PL_Channelizer/LIFO ==
  note: delay valid data output by 1 cycle of count value + 2
  note: ping msb bit
  note: address counts up
  note: ping pong memory configuration
  note: address counts down
  note: pong msb bit
  tvalid_in : Inport
  tdata_in : Inport  Port=2
  Concat : hdlBasic/Concat  num_inputs=2  XmcBlockStatus=1  maskContainerNames=group1  block_type=concat  block_config=sysgen:Concat_config
  Concat2 : hdlBasic/Concat  num_inputs=2  XmcBlockStatus=1  maskContainerNames=group1  block_type=concat  block_config=sysgen:Concat_config
  Constant : hdlBasic/Constant  const=flip_cnt  gui_display_data_type=Fixed-point  arith_type=Unsigned  n_bits=ceil(log2(flip_cnt))  bin_pt=0  preci_type=Single  exp_width=8  frac_width=24  explicit_period=off  period=1  XmcBlockStatus=1  maskContainerNames=tabcontainer1  block_type=constant  block_config=sysgen:Constant_config
  Constant2 : hdlBasic/Constant  const=0  gui_display_data_type=Boolean  arith_type=Boolean  n_bits=16  bin_pt=14  preci_type=Single  exp_width=8  frac_width=24  explicit_period=off  period=1  XmcBlockStatus=1  maskContainerNames=tabcontainer1  block_type=constant  block_config=sysgen:Constant_config
  Constant3 : hdlBasic/Constant  const=0  gui_display_data_type=Fixed-point  arith_type=Unsigned  n_bits=23  bin_pt=22  preci_type=Single  exp_width=8  frac_width=24  explicit_period=off  period=1  XmcBlockStatus=1  maskContainerNames=tabcontainer1  block_type=constant  block_config=sysgen:Constant_config
  Counter : hdlBasic/Counter  cnt_type=Count limited  cnt_to=flip_cnt  operation=Up  start_count=0  cnt_by_val=1  arith_type=Unsigned  n_bits=ceil(log2(flip_cnt))  bin_pt=0  load_pin=off  rst=off  en=on  explicit_period=Inferred from inputs  period=1  use_behavioral_HDL=off  implementation=Fabric  XmcBlockStatus=1  maskContainerNames=group1  block_type=counter  block_config=sysgen:Counter_config  block_width=531  block_height=1023
  Counter1 : hdlBasic/Counter  cnt_type=Free running  cnt_to=Inf  operation=Up  start_count=0  cnt_by_val=1  arith_type=Unsigned  n_bits=1  bin_pt=0  load_pin=off  rst=off  en=on  explicit_period=Inferred from inputs  period=1  use_behavioral_HDL=off  implementation=Fabric  XmcBlockStatus=1  maskContainerNames=group1  block_type=counter  block_config=sysgen:Counter_config  block_width=531  block_height=1023
  Counter3 : hdlBasic/Counter  cnt_type=Count limited  cnt_to=0  operation=Down  start_count=flip_cnt  cnt_by_val=1  arith_type=Unsigned  n_bits=ceil(log2(flip_cnt))  bin_pt=0  load_pin=off  rst=off  en=on  explicit_period=Inferred from inputs  period=1  use_behavioral_HDL=off  implementation=Fabric  XmcBlockStatus=1  maskContainerNames=group1  block_type=counter  block_config=sysgen:Counter_config  block_width=531  block_height=1023
  Delay2 : hdlBasic/Delay  rst=off  en=off  latency=flip_cnt+2  reg_retiming=off  XmcBlockStatus=1  maskContainerNames=group1  block_type=delay  block_config=sysgen:Delay_config
  Dual Port RAM : hdlBasic/Dual Port RAM  depth=2^(ceil(log2(flip_cnt)+1))  initVector=zeros(2^(ceil(log2(flip_cnt)+1)))  distributed_mem=Block RAM  init_a=0  init_b=0  rst_a=off  rst_b=off  en_a=off  en_b=off  latency=1  write_mode_A=Read After Write  write_mode_B=Read After Write  explicit_period=[]  period=[]  simulation_type=fast_sim  XmcBlockStatus=1  maskContainerNames=tabcontainer1  block_type=dpram  block_config=sysgen:Dpram_config  optimize=Area
      settings: infoedit=[]
  Inverter1 : hdlBasic/Inverter  en=off  latency=0  XmcBlockStatus=1  maskContainerNames=group2  block_type=inv  block_config=sysgen:Inverter_config
  Relational : hdlBasic/Relational  mode=a=b  op_type=Bool  en=off  latency=0  XmcBlockStatus=1  maskContainerNames=tabcontainer1  block_type=relational  block_config=sysgen:Relational_config
  Terminator : Terminator
  tdata_out : Outport
  tvalid_out : Outport  Port=2
  wires:
  Constant3/1 -> Dual Port RAM/5
  Relational/1 -> Counter1/1
  Constant2/1 -> Dual Port RAM/6
  Concat/1 -> Dual Port RAM/1  "addra"
  Counter/1 -> Relational/2, Concat/2  "lsb"
  Delay2/1 -> tvalid_out/1  "tvalid_out"
  Constant/1 -> Relational/1
  Dual Port RAM/2 -> tdata_out/1  "tdata_out"
  tvalid_in/1 -> Counter3/1, Counter/1, Dual Port RAM/3, Delay2/1  "tvalid_in"
  Dual Port RAM/1 -> Terminator/1
  Counter1/1 -> Inverter1/1, Concat/1  "msb"
  Inverter1/1 -> Concat2/1  "msb_addrb"
  Counter3/1 -> Concat2/2  "lsb_addrb"
  Concat2/1 -> Dual Port RAM/4  "concat_addrb"
  tdata_in/1 -> Dual Port RAM/2  "tdata_in"

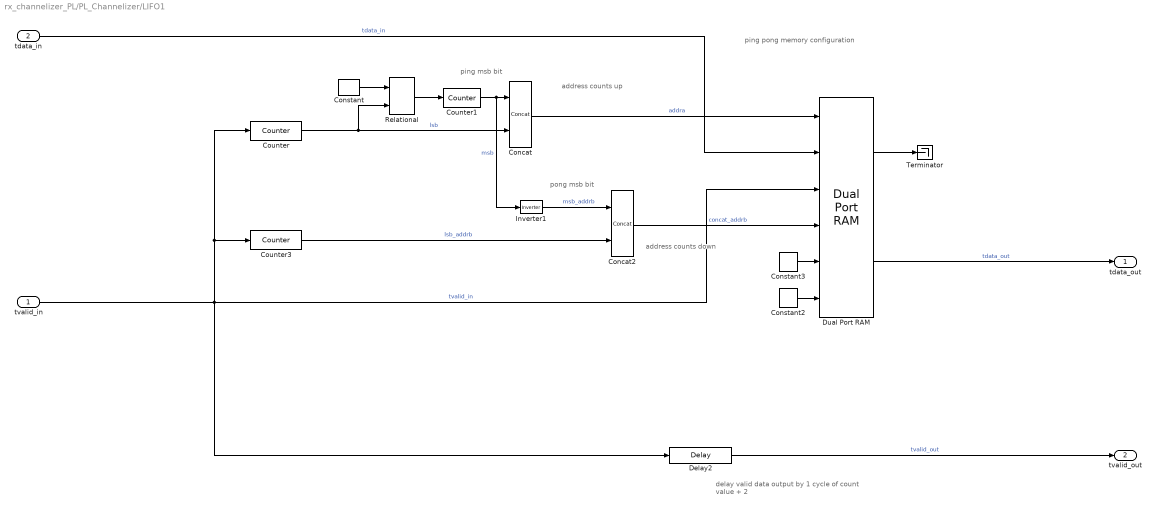
== system rx_channelizer_PL/PL_Channelizer/LIFO1 ==
  note: pong msb bit
  note: address counts down
  note: ping pong memory configuration
  note: address counts up
  note: ping msb bit
  note: delay valid data output by 1 cycle of count value + 2
  tvalid_in : Inport
  tdata_in : Inport  Port=2
  Concat : hdlBasic/Concat  num_inputs=2  XmcBlockStatus=1  maskContainerNames=group1  block_type=concat  block_config=sysgen:Concat_config
  Concat2 : hdlBasic/Concat  num_inputs=2  XmcBlockStatus=1  maskContainerNames=group1  block_type=concat  block_config=sysgen:Concat_config
  Constant : hdlBasic/Constant  const=flip_cnt  gui_display_data_type=Fixed-point  arith_type=Unsigned  n_bits=ceil(log2(flip_cnt))  bin_pt=0  preci_type=Single  exp_width=8  frac_width=24  explicit_period=off  period=1  XmcBlockStatus=1  maskContainerNames=tabcontainer1  block_type=constant  block_config=sysgen:Constant_config
  Constant2 : hdlBasic/Constant  const=0  gui_display_data_type=Boolean  arith_type=Boolean  n_bits=16  bin_pt=14  preci_type=Single  exp_width=8  frac_width=24  explicit_period=off  period=1  XmcBlockStatus=1  maskContainerNames=tabcontainer1  block_type=constant  block_config=sysgen:Constant_config
  Constant3 : hdlBasic/Constant  const=0  gui_display_data_type=Fixed-point  arith_type=Unsigned  n_bits=23  bin_pt=22  preci_type=Single  exp_width=8  frac_width=24  explicit_period=off  period=1  XmcBlockStatus=1  maskContainerNames=tabcontainer1  block_type=constant  block_config=sysgen:Constant_config
  Counter : hdlBasic/Counter  cnt_type=Count limited  cnt_to=flip_cnt  operation=Up  start_count=0  cnt_by_val=1  arith_type=Unsigned  n_bits=ceil(log2(flip_cnt))  bin_pt=0  load_pin=off  rst=off  en=on  explicit_period=Inferred from inputs  period=1  use_behavioral_HDL=off  implementation=Fabric  XmcBlockStatus=1  maskContainerNames=group1  block_type=counter  block_config=sysgen:Counter_config  block_width=531  block_height=1023
  Counter1 : hdlBasic/Counter  cnt_type=Free running  cnt_to=Inf  operation=Up  start_count=0  cnt_by_val=1  arith_type=Unsigned  n_bits=1  bin_pt=0  load_pin=off  rst=off  en=on  explicit_period=Inferred from inputs  period=1  use_behavioral_HDL=off  implementation=Fabric  XmcBlockStatus=1  maskContainerNames=group1  block_type=counter  block_config=sysgen:Counter_config  block_width=531  block_height=1023
  Counter3 : hdlBasic/Counter  cnt_type=Count limited  cnt_to=0  operation=Down  start_count=flip_cnt  cnt_by_val=1  arith_type=Unsigned  n_bits=ceil(log2(flip_cnt))  bin_pt=0  load_pin=off  rst=off  en=on  explicit_period=Inferred from inputs  period=1  use_behavioral_HDL=off  implementation=Fabric  XmcBlockStatus=1  maskContainerNames=group1  block_type=counter  block_config=sysgen:Counter_config  block_width=531  block_height=1023
  Delay2 : hdlBasic/Delay  rst=off  en=off  latency=flip_cnt+2  reg_retiming=off  XmcBlockStatus=1  maskContainerNames=group1  block_type=delay  block_config=sysgen:Delay_config
  Dual Port RAM : hdlBasic/Dual Port RAM  depth=2^(ceil(log2(flip_cnt)+1))  initVector=zeros(2^(ceil(log2(flip_cnt)+1)))  distributed_mem=Block RAM  init_a=0  init_b=0  rst_a=off  rst_b=off  en_a=off  en_b=off  latency=1  write_mode_A=Read After Write  write_mode_B=Read After Write  explicit_period=[]  period=[]  simulation_type=fast_sim  XmcBlockStatus=1  maskContainerNames=tabcontainer1  block_type=dpram  block_config=sysgen:Dpram_config  optimize=Area
      settings: infoedit=[]
  Inverter1 : hdlBasic/Inverter  en=off  latency=0  XmcBlockStatus=1  maskContainerNames=group2  block_type=inv  block_config=sysgen:Inverter_config
  Relational : hdlBasic/Relational  mode=a=b  op_type=Bool  en=off  latency=0  XmcBlockStatus=1  maskContainerNames=tabcontainer1  block_type=relational  block_config=sysgen:Relational_config
  Terminator : Terminator
  tdata_out : Outport
  tvalid_out : Outport  Port=2
  wires:
  tdata_in/1 -> Dual Port RAM/2  "tdata_in"
  Concat2/1 -> Dual Port RAM/4  "concat_addrb"
  Counter3/1 -> Concat2/2  "lsb_addrb"
  Inverter1/1 -> Concat2/1  "msb_addrb"
  Counter1/1 -> Concat/1, Inverter1/1  "msb"
  Dual Port RAM/1 -> Terminator/1
  tvalid_in/1 -> Delay2/1, Dual Port RAM/3, Counter/1, Counter3/1  "tvalid_in"
  Dual Port RAM/2 -> tdata_out/1  "tdata_out"
  Constant/1 -> Relational/1
  Delay2/1 -> tvalid_out/1  "tvalid_out"
  Counter/1 -> Concat/2, Relational/2  "lsb"
  Concat/1 -> Dual Port RAM/1  "addra"
  Constant2/1 -> Dual Port RAM/6
  Relational/1 -> Counter1/1
  Constant3/1 -> Dual Port RAM/5
